simulink model "FluxModel2015a_verify_Q_zhixin"  (R2020b)
settings: Solver=VariableStepAuto  StartTime=0.0  StopTime=0.3  FixedStep=Ts  RelTol=1e-3  EnableMultiTasking=on
model workspace (MAT data in the model file):
  MOVE : Simulink.Parameter (value not decoded)
  STOP : Simulink.Parameter (value not decoded)
  thres : Simulink.Parameter (value not decoded)
values from neighbouring files (symbols this model uses):
  AngleEncoderEn = 1    [parameters.m]
  AngleSpdClosedLoopEnable = 0.0    (= 0)    [parameters.m]
  CurrentLoopMax = Q14*1.2    (= 19660.8)    [parameters.m]
  EstOutMax_Speed_Q = Q14*1.2    (= 19660.8)    [parameters.m]
  Factor1 = Q15*Ts*Rb/Lq_realvalue    [parameters.m]
  Factor2 = Q15*Ts*Rs_realvalue/Lq_realvalue    (= 16990.2962963)    [parameters.m]
  fieldweaken_Max = 0    [parameters.m]
  fieldweaken_Min = -0.5*Q14    (= -8192)    [parameters.m]
  FieldWeakenEn = 0    [parameters.m]
  fluxF = Lam_realvalue/fluxB    [parameters.m]
  fluxF_Q14 = Q14*fluxF    [parameters.m]
  Friction = 0.003    [parameters.m]
  Ib = sqrt(2)*In    [parameters.m]
  Id_Ki = Q14*CurrentLoopBandwidth*Rs    [parameters.m]
  Id_Kp = Q14*CurrentLoopBandwidth*Ld    [parameters.m]
  IFCurrDecreased = 1    [parameters.m]
  IFCurrStart = 8    [parameters.m]
  IFCurrTarget = 5    [parameters.m]
  IFIdref = 0    [parameters.m]
  initial_degree = 0    [parameters.m]
  Iq_Ki = Q14*CurrentLoopBandwidth*Rs    [parameters.m]
  Iq_Kp = Q14*CurrentLoopBandwidth*Lq    [parameters.m]
  J_realvalue = 2.47e-4    (= 0.000247)    [parameters.m]
  KI_fieldweaken = 0.1*Q14    (= 1638.4)    [parameters.m]
  KP_fieldweaken = 1.0*Q14    (= 16384)    [parameters.m]
  LamObserverGain_Q = Q15*LamObserverGain    (= 13106.8)    [parameters.m]
  Ld = Ld_realvalue/Lb    [parameters.m]
  Ld_Q14 = Q14*Ld_realvalue/Lb    [parameters.m]
  Ld_realvalue = 2.7e-3    (= 0.0027)    [parameters.m]
  LowPassFilterBandWidth_Emf_Q = Q14*LowPassFilterBandWidth_Emf    (= 1445.64705882)    [parameters.m]
  LowPassFilterCoeff_Emf = Q15*(1/(1+LowPassFilterBandWidth_Emf*TsPu))    (= 31292.3812732)    [parameters.m]
  LowPassFilterCoeff_Spd = Q15*(1/(1+LowPassFilterBandWidth_Speed*SpeedloopTs/tb))    (= 20123.2126159)    [parameters.m]
  Lq = Lq_realvalue/Lb    [parameters.m]
  Lq_Q14 = Q14*Lq_realvalue/Lb    [parameters.m]
  Lq_realvalue = 2.7e-3    (= 0.0027)    [parameters.m]
  MOVE = 1    [parameters.m]
  Np = 1    [parameters.m]
  Omega0_Q = Q14*Omega0    (= 6553.6)    [parameters.m]
  OverModulationEn = 0    [parameters.m]
  PLL_KI = Q14*PLL_Bandwidth*PLL_Bandwidth    (= 56.6920415225)    [parameters.m]
  PLL_KP = Q14*2*PLL_Bandwidth    (= 1927.52941176)    [parameters.m]
  PLL_OUTMax_W = Q14*1.2    (= 19660.8)    [parameters.m]
  PWM_Period = 1000    [parameters.m]
  Q14 = 16384    [parameters.m]
  Q15 = 32767    [parameters.m]
  Q16 = 65535    [parameters.m]
  Rs = Rs_realvalue/Rb    [parameters.m]
  Rs_Q14 = Q14*Rs_realvalue/Rb    [parameters.m]
  Rs_realvalue = 28    [parameters.m]
  SecondOverMod = 0    [parameters.m]
  SMO_Gain = Q14*0.85    (= 13926.4)    [parameters.m]
  SMO_I_ERROR = Q14*0.05    (= 819.2)    [parameters.m]
  SpdClosedLoopEnable = 0.0    (= 0)    [parameters.m]
  Speed_Ki = Q14*SpeedLoopBandwidth    (= 481.882352941)    [parameters.m]
  Speed_Kp = Q14*SpeedLoopBandwidth*JPu/fluxF    [parameters.m]
  SpeedIncreased = 0.1*Wb    (= 1068.14150222)    [parameters.m]
  SpeedloopTs = 1/SpeedloopFrequency    (= 0.001)    [parameters.m]
  Speedn = 60*fn/Np    (= 102000)    [parameters.m]
  SpeedOutmax = 1.2*Q14    (= 19660.8)    [parameters.m]
  SpeedSwitch = 0.6*Wb    (= 6408.84901332)    [parameters.m]
  SpeedTarget = 0.8*Wb    (= 8545.13201776)    [parameters.m]
  STOP = 0    [parameters.m]
  SVCM_GAIN_Q = Q15*SVCM_GAIN    (= 26213.6)    [parameters.m]
  tb = 1/Wb    (= 9.36205547599e-05)    [parameters.m]
  Tf = 0    [parameters.m]
  thres = 0.1    [parameters.m]
  Tn = 0.012    [parameters.m]
  Ts = 1/SwitchFrequency    (= 5e-05)    [parameters.m]
  TsPu = Ts/tb    (= 0.53407075111)    [parameters.m]
  Vb = Vdc/sqrt(3)    [parameters.m]
  Vdc = sqrt(2)*Un    [parameters.m]
  Wb = 2*pi*fn    (= 10681.4150222)    [parameters.m]
  ZeroSeqInjectEn = 0.0    (= 0)    [parameters.m]
undefined symbols (not defined in the file or in its folder): DiscIntNeverNeededParam, EstOutMax_Theta, magnitude, sigbuilder_block
libraries: simulink x9, powerlib x5, mcbutilslib x1
(part 3 of 3)

== system FluxModel2015a_verify_Q_zhixin/CurrLoop&Observer/SVCM/park1 ==
  alpha : Inport
  beta : Inport  Port=2
  theta : Inport  Port=3
  Add : Sum
  Add1 : Sum  Inputs=+-
  Product{,1..3} (4 alike) : Product
  Sin : Trigonometry
  Sin1 : Trigonometry  Operator=cos
  D : Outport
  Q : Outport  Port=2
  wires:
  Add1/1 -> Q/1
  alpha/1 -> Product/1, Product3/1
  Product/1 -> Add/1
  Product1/1 -> Add/2
  beta/1 -> Product2/1, Product1/1
  Sin1/1 -> Product/2, Product2/2
  Product3/1 -> Add1/2
  Add/1 -> D/1
  Sin/1 -> Product1/2, Product3/2
  Product2/1 -> Add1/1
  theta/1 -> Sin/1, Sin1/1

== system FluxModel2015a_verify_Q_zhixin/SVPWM/VoltReconstruct/Subsystem6 ==
  CCR1 : Inport
  Add : Sum  Inputs=+-
  Constant1 : Constant  Value=Ts/2
  Divide : Product  Inputs=/*
  Product : Product
  Vdc1 : Constant  Value=Vdc
  Uao : Outport
  wires:
  Constant1/1 -> Divide/1, Add/1
  Product/1 -> Uao/1
  CCR1/1 -> Add/2
  Add/1 -> Divide/2
  Divide/1 -> Product/2
  Vdc1/1 -> Product/1

== system FluxModel2015a_verify_Q_zhixin/SVPWM/VoltReconstruct/Subsystem7 ==
  CCR2 : Inport
  Add : Sum  Inputs=+-
  Constant1 : Constant  Value=Ts/2
  Divide : Product  Inputs=/*
  Product : Product
  Vdc1 : Constant  Value=Vdc
  Ubo : Outport
  wires:
  Constant1/1 -> Divide/1, Add/1
  Product/1 -> Ubo/1
  CCR2/1 -> Add/2
  Add/1 -> Divide/2
  Divide/1 -> Product/2
  Vdc1/1 -> Product/1

== system FluxModel2015a_verify_Q_zhixin/SVPWM/VoltReconstruct/Subsystem8 ==
  CCR3 : Inport
  Add : Sum  Inputs=+-
  Constant1 : Constant  Value=Ts/2
  Divide : Product  Inputs=/*
  Product : Product
  Vdc1 : Constant  Value=Vdc
  Uco : Outport
  wires:
  Constant1/1 -> Divide/1, Add/1
  Product/1 -> Uco/1
  CCR3/1 -> Add/2
  Add/1 -> Divide/2
  Divide/1 -> Product/2
  Vdc1/1 -> Product/1

== matlab function FluxModel2015a_verify_Q_zhixin/SVPWM/MATLAB Function1 ==
  data: T1 input; y1 output; T2 input; Ts input; y2 output
function [y1,y2] = fcn(T1,T2,Ts)
if (T1+T2) > Ts
    T1 = T1*Ts/(T1+T2);
    T2 = T2*Ts/(T1+T2);
end
y1 = T1;
y2 = T2;
end

== matlab function FluxModel2015a_verify_Q_zhixin/SVPWM/MATLAB Function ==
  data: T1 input; y1 output; T2 input; y2 output; Ts input; Tsum data_store_memory; Tdelt data_store_memory
function [y1,y2] = fcn(T1,T2,Ts)
global Tsum;
global Tdelt;
Tsum = T1+T2;
if Tsum > Ts
    T1 = T1*Ts/Tsum;
    T2 = T2*Ts/Tsum;
end
if Tsum > 1.154*Ts
   Tdelt = 1.154*Ts - Tsum;
   if T1 > T2
       if T2 < Tdelt
           T2 = 0;
           T1 = Ts;
       else
           T2 = T2 - Tdelt;
           T1 = T1 + Tdelt;
       end
   else
       if T1 < Tdelt
           T1 = 0;
           T2 = Ts;
       else
           T1 = T1 - Tdelt;
           T2 = T2 + Tdelt;
       end
   end
end

y1 = T1;
y2 = T2;        
end

== stateflow chart FluxModel2015a_verify_Q_zhixin/Chart ==
  settings: executeAtInitialization=1
  state STOP
    en:
    MotionState = STOP;
    du:
    MotionState = STOP;
  state Move
    en:
    MotionState = MOVE;
    du:
    MotionState = MOVE;
  (default) -> STOP
  STOP -> Move : [Speed>=thres]
  Move -> STOP : [Speed<thres]
  data: Speed input double; MotionState output boolean; STOP parameter; MOVE parameter; thres parameter

== matlab function FluxModel2015a_verify_Q_zhixin/SVPWM/MATLAB Function2 ==
  data: T1 input; y1 output; T2 input; Ts input; y2 output
function [y1,y2] = fcn(T1,T2,Ts)
if (T1+T2) > Ts
    T1 = T1*Ts/(T1+T2);
    T2 = T2*Ts/(T1+T2);
end
y1 = T1;
y2 = T2;
end

== matlab function FluxModel2015a_verify_Q_zhixin/Note/MATLAB Function ==
  data: u input; y output
function y = fcn(u)

y = u;
